simulink model "gyroSystem"  (R2019a)
settings: Solver=VariableStepAuto  StartTime=0.0  StopTime=10.0  RelTol=1e-3
settings Model: Creator=Dario Quintero  LastModifiedBy=dq16394
settings DebuggingCC: PregeneratedLibrarySubsystemCodeDiagnostic=none  ArithmeticOperatorsInVariantConditions=warning

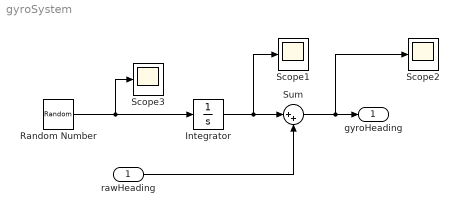
== system gyroSystem ==
  rawHeading : Inport
  Integrator : Integrator
  Random Number : RandomNumber  Mean=0.02  Variance=0.01  SampleTime=0.1
  Scope1 : Scope
  Scope2 : Scope
  Scope3 : Scope
  Sum : Sum  Inputs=|++
  gyroHeading : Outport
  wires:
  Random Number/1 -> Scope3/1, Integrator/1
  Integrator/1 -> Scope1/1, Sum/1
  rawHeading/1 -> Sum/2
  Sum/1 -> Scope2/1, gyroHeading/1
